simulink library "ESTS_FRIC_HILO_LIM"  (R2024b)
settings: Solver=VariableStepAuto  StartTime=0.0  StopTime=10.0  RelTol=1e-3
undefined symbols (not defined in the file): ESTS_FRIC_HILO_LIM_p_MaxFricLoMue_na, ESTS_FRIC_HILO_LIM_p_MinFricHiMue_na, ESTS_FRIC_HILO_LIM_p_TqMaxLoMueMax_Nm, ESTS_FRIC_HILO_LIM_p_TqMaxLoMueMin_Nm, ESTS_FRIC_HILO_LIM_p_TqMinHiMueMax_Nm, ESTS_FRIC_HILO_LIM_p_TqMinHiMueMin_Nm, p_RadWhlDynFr_m, p_RadWhlDynRe_m
libraries: simulink x2
settings Model: Creator=blatak  LastModifiedBy=blatak

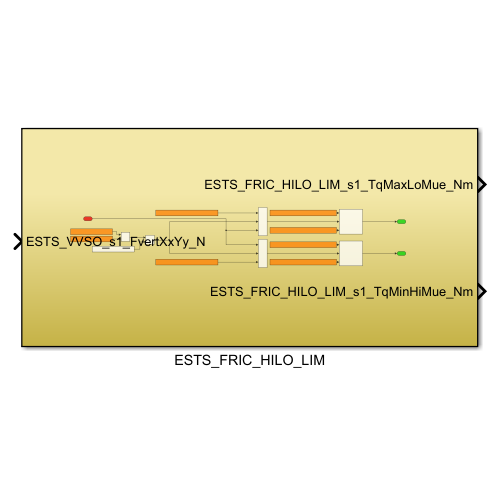
[thumbnail: Simulink's stored preview of the top-level diagram]
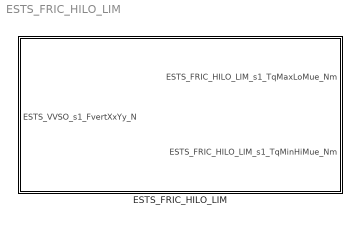
== system ESTS_FRIC_HILO_LIM ==
  ESTS_FRIC_HILO_LIM : Subsystem

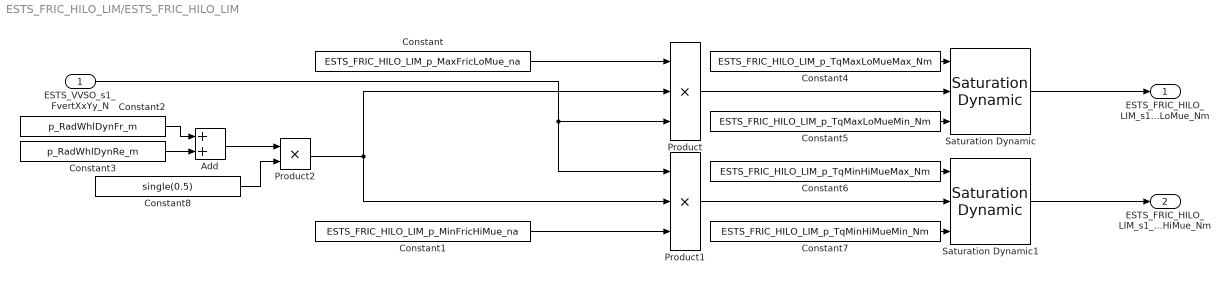
== system ESTS_FRIC_HILO_LIM/ESTS_FRIC_HILO_LIM ==
  ESTS_VVSO_s1_FvertXxYy_N : Inport
  Add : Sum
  Constant : Constant  Value=ESTS_FRIC_HILO_LIM_p_MaxFricLoMue_na
  Constant1 : Constant  Value=ESTS_FRIC_HILO_LIM_p_MinFricHiMue_na
  Constant2 : Constant  Value=p_RadWhlDynFr_m
  Constant3 : Constant  Value=p_RadWhlDynRe_m
  Constant4 : Constant  Value=ESTS_FRIC_HILO_LIM_p_TqMaxLoMueMax_Nm
  Constant5 : Constant  Value=ESTS_FRIC_HILO_LIM_p_TqMaxLoMueMin_Nm
  Constant6 : Constant  Value=ESTS_FRIC_HILO_LIM_p_TqMinHiMueMax_Nm
  Constant7 : Constant  Value=ESTS_FRIC_HILO_LIM_p_TqMinHiMueMin_Nm
  Constant8 : Constant  Value=single(0.5)
  Product : Product  Inputs=3
  Product1 : Product  Inputs=3
  Product2 : Product
  Saturation Dynamic : simulink/Discontinuities/Saturation Dynamic  OutMin=[]  OutMax=[]  OutDataTypeStr=Inherit: Same as second input  OutDataType=fixdt(1, 16)  OutScaling=2^-10  DoSatur=off
  Saturation Dynamic1 : simulink/Discontinuities/Saturation Dynamic  OutMin=[]  OutMax=[]  OutDataTypeStr=Inherit: Same as second input  OutDataType=fixdt(1, 16)  OutScaling=2^-10  DoSatur=off
  ESTS_FRIC_HILO_LIM_s1_TqMaxLoMue_Nm : Outport
  ESTS_FRIC_HILO_LIM_s1_TqMinHiMue_Nm : Outport  Port=2
  wires:
  Product/1 -> Saturation Dynamic/2
  Constant8/1 -> Product2/2
  ESTS_VVSO_s1_FvertXxYy_N/1 -> Product1/1, Product/3
  Constant6/1 -> Saturation Dynamic1/1
  Product2/1 -> Product/2, Product1/2
  Constant2/1 -> Add/1
  Constant1/1 -> Product1/3
  Constant/1 -> Product/1
  Saturation Dynamic/1 -> ESTS_FRIC_HILO_LIM_s1_TqMaxLoMue_Nm/1
  Constant5/1 -> Saturation Dynamic/3
  Saturation Dynamic1/1 -> ESTS_FRIC_HILO_LIM_s1_TqMinHiMue_Nm/1
  Product1/1 -> Saturation Dynamic1/2
  Add/1 -> Product2/1
  Constant7/1 -> Saturation Dynamic1/3
  Constant3/1 -> Add/2
  Constant4/1 -> Saturation Dynamic/1
